simulink model "untitled"  (R2015a)
settings: Solver=ode45  StartTime=0.0  StopTime=0  RelTol=1e-3
undefined symbols (not defined in the file or in its folder): gray, jet
libraries: visionsinks x4, visionsources x1
settings Model: Creator=Sparsh-PC  LastModifiedBy=Sparsh-PC

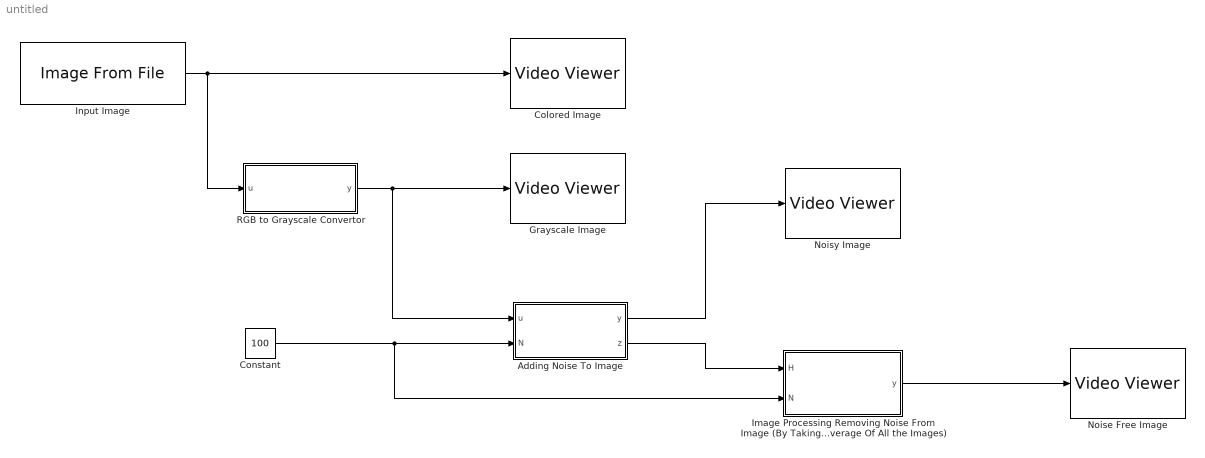
== system untitled ==
  Adding Noise To Image : MATLAB Function  TreatAsAtomicUnit=on
  Colored Image : visionsinks/Video Viewer  inputType=Obsolete7b  imagePorts=One multidimensional signal  useColorMap=off  colormapValue=gray(256)  specRange=off  minInputVal=0  maxInputVal=255  FigPos=[727 799 410 300]  AxisZoom=on  trueSizedOnce=off  OpenAtMdlStart=on  DefaultConfigurationName=vipscopes.VideoViewerScopeCfg
  Constant : Constant  Value=100  SampleTime=0  LockScale=on
  Grayscale Image : visionsinks/Video Viewer  inputType=Obsolete7b  imagePorts=One multidimensional signal  useColorMap=off  colormapValue=jet(256)  specRange=off  minInputVal=0  maxInputVal=255  FigPos=[722 657 410 294]  AxisZoom=on  trueSizedOnce=off  OpenAtMdlStart=on  DefaultConfigurationName=vipscopes.VideoViewerScopeCfg
  Image Processing Removing Noise From Image (By Taking Average Of All the Images) : MATLAB Function  TreatAsAtomicUnit=on
  Input Image : visionsources/Image From File  Tag=vipblks_nd  FileName=img.jpg  imagePorts=One multidimensional signal  Ts=inf  ImageDataType=Inherit from input image  Signed=on  WordLength=16  sdImageDataType=uint(8)  FractionLengthMode=User-defined  FractionLength=15  OutPortLabels=R|G|B
  Noise Free Image : visionsinks/Video Viewer  inputType=Obsolete7b  imagePorts=One multidimensional signal  useColorMap=off  colormapValue=jet(256)  specRange=off  minInputVal=0  maxInputVal=255  FigPos=[126 674 410 300]  AxisZoom=on  trueSizedOnce=off  OpenAtMdlStart=on  DefaultConfigurationName=vipscopes.VideoViewerScopeCfg
  Noisy Image : visionsinks/Video Viewer  inputType=Obsolete7b  imagePorts=One multidimensional signal  useColorMap=off  colormapValue=jet(256)  specRange=off  minInputVal=0  maxInputVal=255  FigPos=[518 692 410 300]  AxisZoom=on  trueSizedOnce=off  OpenAtMdlStart=on  DefaultConfigurationName=vipscopes.VideoViewerScopeCfg
  RGB to Grayscale Convertor : MATLAB Function  TreatAsAtomicUnit=on
  wires:
  Input Image/1 -> Colored Image/1, RGB to Grayscale Convertor/1(u)
  Adding Noise To Image/1(y) -> Noisy Image/1
  RGB to Grayscale Convertor/1(y) -> Adding Noise To Image/1(u), Grayscale Image/1
  Constant/1 -> Image Processing Removing Noise From Image (By Taking Average Of All the Images)/2(N), Adding Noise To Image/2(N)
  Adding Noise To Image/2(z) -> Image Processing Removing Noise From Image (By Taking Average Of All the Images)/1(H)
  Image Processing Removing Noise From Image (By Taking Average Of All the Images)/1(y) -> Noise Free Image/1

== matlab function untitled/Adding Noise To Image ==
  data: u input; y output; N input; z output
function [y,z]= AddNoise(u,N)
mean = 0.0; 
var = 0.0887;
dim = 500;
w = zeros(225*dim,225);

J = im2double(u);
b = (J + rand(size(J))*sqrt(var) + mean);
%b = (imnoise(J,'gaussian',0,0.458));
%b = (imnoise(J,'salt & pepper',0.05));
%b = (imnoise(J,'poisson'));

for i=1:N
    w(225*(i-1)+1:225*(i-1)+225,:) = (J + rand(size(J))*sqrt(var) + mean);
end;
y = b;
z = w;

== matlab function untitled/RGB to Grayscale Convertor ==
  data: u input; y output
function y = RGBtoGrayImage(u)
y = rgb2gray(u);

== matlab function untitled/Image Processing Removing Noise From Image (By Taking Average Of All the Images) ==
  data: H input; y output; N input
function y = RemoveNoise(H,N)
sum = zeros(225,225);
for i=1:N
   sum = sum + (H(225*(i-1)+1:225*(i-1)+225,:)/N);
end;
y = sum;
